simulink model "simulacao_ss_compatibilidade"  (Simulink 7.7)
settings: Solver=ode3  SolverMode=SingleTasking  StartTime=0.0  StopTime=10.0  FixedStep=0.0001  RelTol=1e-3
values from neighbouring files (symbols this model uses):
  Ki = Kext(3)    [MDLsspace.m]    (also in dadosSS.mat = 0.0705482633825; dadosSS3.mat = -0.00217932892475; ssGera.m = Kext(4))
  Kproc = [Kext(1), Kext(2)]    [MDLsspace.m]    (also in dadosSS.mat = [-8.78793449987 -65.7586899975]; dadosSS3.mat = [-634.744698351 -20071.4503166 -147729.126991]; ssGera.m = [Kext(1), Kext(2), Kext(3)])
  L = (acker(A', C', polosObs))'    [MDLsspace.m]    (also in dadosSS.mat = [0.0267900926393 -0.00885593505471]; dadosSS3.mat = [-62.4863664427 0.0974835238697 -0.000151272035649]; ssGera.m)
settings Model: Creator=root  LastModifiedBy=root  CovMetricSettings=dwe  CovHtmlReporting=off  covSaveCumulativeToWorkspaceVar=off  CovSaveSingleToWorkspaceVar=off  CovExternalEMLEnable=on
settings SolverCC: ZeroCrossAlgorithm=Adaptive
settings DataIOCC: LimitDataPoints=off  SaveFormat=StructureWithTime  SignalLoggingSaveFormat=Dataset
settings OptimizationCC: ExpressionDepthLimit=128
settings DebuggingCC: UnderspecifiedInitializationDetection=Simplified  MergeDetectMultiDrivingBlocksExec=error  MaxConsecutiveZCsMsg=none  SolverPrmCheckMsg=none  FcnCallInpInsideContextMsg=Enable All  StateNameClashWarn=none  SFUnexpectedBacktrackingDiag=error  SFNoUnconditionalDefaultTransitionDiag=error
settings HardwareCC: ProdBitPerPointer=64  ProdLargestAtomicFloat=Float  ProdIntDivRoundTo=Zero  ProdEndianess=LittleEndian  ProdHWDeviceType=Specified
settings CodeAppCC: CustomSymbolStrType=$N$R$M_T
settings GRTTargetCC: TargetFunctionLibrary=C99 (ISO)  GeneratePreprocessorConditionals=Use local settings

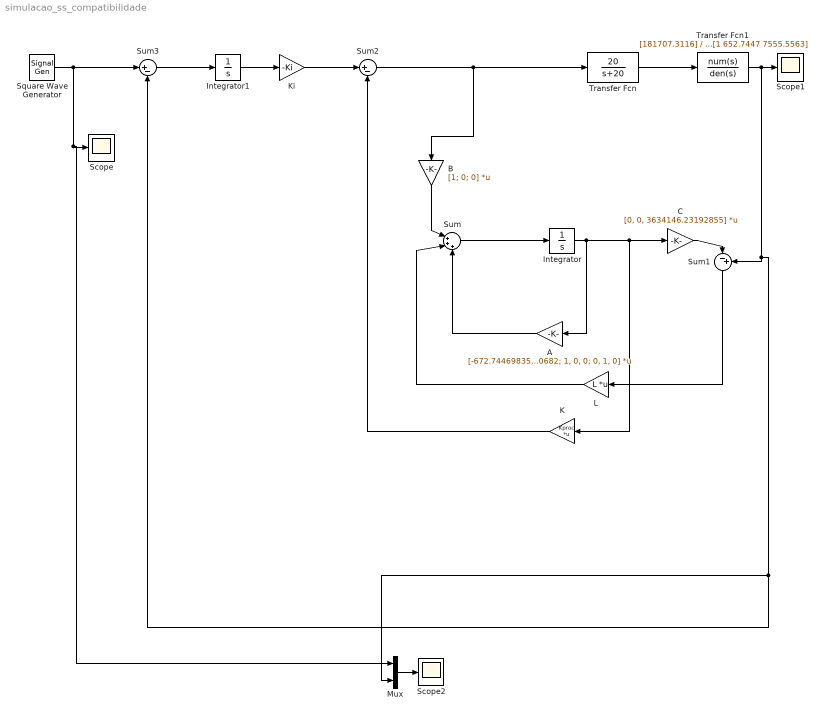
== system simulacao_ss_compatibilidade ==
  A : Gain  Gain="[-672.744698351479,  -20610.4503165634, -151111.126990682; 1, 0, 0; 0, 1, 0]"  Multiplication=Matrix(K*u)
  B : Gain  Gain=[1; 0; 0]  Multiplication=Matrix(K*u)
  C : Gain  Gain=[0, 0, 3634146.23192855]  Multiplication=Matrix(K*u)
  Integrator : Integrator
  Integrator1 : Integrator
  K : Gain  Gain=Kproc  Multiplication=Matrix(K*u)
  Ki : Gain  Gain=-Ki
  L : Gain  Gain=L  Multiplication=Matrix(K*u)
  Mux : Mux  Inputs=2
  Scope : Scope
      settings: TimeRange=auto  MaxDataPoints=5000  SaveToWorkspace=off  SaveName=ScopeData  YMin=-56.25  YMax=56.25  SampleTime=-1
  Scope1 : Scope
      settings: TimeRange=auto  MaxDataPoints=5000  SaveToWorkspace=off  YMin=-56.25  YMax=56.25  SampleTime=-1
  Scope2 : Scope
      settings: TimeRange=auto  MaxDataPoints=5000  SaveToWorkspace=off  YMin=-56.25  YMax=56.25  SampleTime=-1
  Square Wave Generator : SignalGenerator  WaveForm=square  Amplitude=45  Units=rad/sec
  Sum : Sum  Inputs=|+++
  Sum1 : Sum  Inputs=|-+
  Sum2 : Sum  Inputs=|+-
  Sum3 : Sum  Inputs=|+-
  Transfer Fcn : TransferFcn  Numerator=[20]  Denominator=[1, 20]
  Transfer Fcn1 : TransferFcn  Numerator=[181707.3116]  Denominator=[1 652.7447 7555.5563]
  wires:
  Sum2/1 -> B/1, Transfer Fcn/1
  Sum/1 -> Integrator/1
  Integrator/1 -> K/1, C/1, A/1
  A/1 -> Sum/3
  C/1 -> Sum1/1
  B/1 -> Sum/1
  Sum1/1 -> L/1
  L/1 -> Sum/2
  K/1 -> Sum2/2
  Integrator1/1 -> Ki/1
  Ki/1 -> Sum2/1
  Transfer Fcn1/1 -> Scope1/1, Mux/2, Sum3/2, Sum1/2
  Sum3/1 -> Integrator1/1
  Square Wave Generator/1 -> Mux/1, Scope/1, Sum3/1
  Transfer Fcn/1 -> Transfer Fcn1/1
  Mux/1 -> Scope2/1
